simulink model "test"  (R2024a)
settings: Solver=VariableStepAuto  StartTime=0.0  StopTime=10.0  RelTol=1e-3
libraries: instrumentlib x2
settings Model: Creator=owenc  LastModifiedBy=owenc
settings RTWCC: GPUComputeCapability=3.5

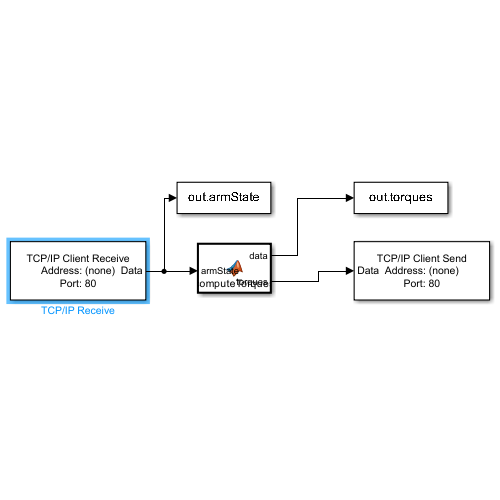
[thumbnail: Simulink's stored preview of the top-level diagram]
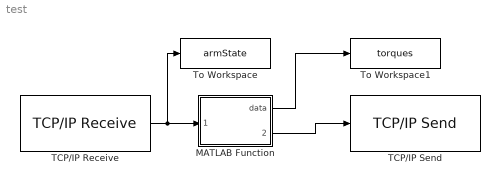
== system test ==
  MATLAB Function : MATLAB Function  TreatAsAtomicUnit=on
  TCP/IP Receive : instrumentlib/TCP//IP Receive  Port=80  DataSize=[ 1, 7 ]  DataType=uint8  ASCIIFormatting=%f  Terminator=LF  CustomTerminator=10  ByteOrder=big-endian  EnableBlockingMode=on  Timeout=10  SampleTime=0.01  SimulateUsing=Interpreted execution
  TCP/IP Send : instrumentlib/TCP//IP Send  Port=80  ByteOrder=big-endian  EnableBlockingMode=on  Timeout=10  TransferDelay=on  SimulateUsing=Interpreted execution
  To Workspace : ToWorkspace  VariableName=armState  SampleTime=-1
  To Workspace1 : ToWorkspace  VariableName=torques  SampleTime=-1
  wires:
  TCP/IP Receive/1 -> To Workspace/1, MATLAB Function/1(armState)
  MATLAB Function/2(torques) -> TCP/IP Send/1
  MATLAB Function/1(data) -> To Workspace1/1

== matlab function test/MATLAB Function ==
  data: data output; armState input; torques output
function [data, torques]= computeTorques(armState)
    torques = armState + 1;
end
